simulink library "flexy_air_lib"  (R2020a)
settings: Solver=VariableStepAuto  StartTime=0.0  StopTime=10.0  RelTol=1e-3
settings Model: Creator=MK  LastModifiedBy=MK

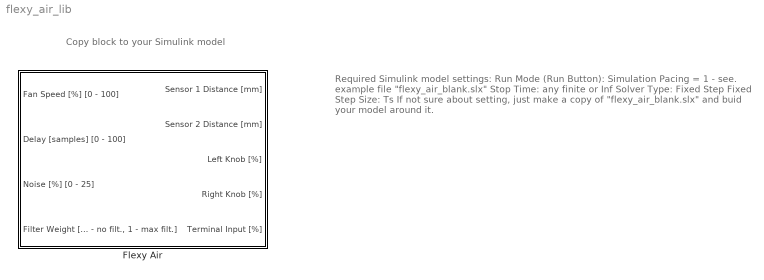
== system flexy_air_lib ==
  note: Copy block to your Simulink model
  note: Required Simulink model settings:
      |
      | Run Mode (Run Button): Simulation Pacing = 1 - see. example file "flexy_air_blank.slx"
      | Stop Time: any finite or Inf
      | Solver Type: Fixed Step
      | Fixed Step Size: Ts
      |
      | If not sure about setting, just make a copy of "flexy_air_blank.slx"
      | and buid your model around it.
  Flexy Air : Subsystem

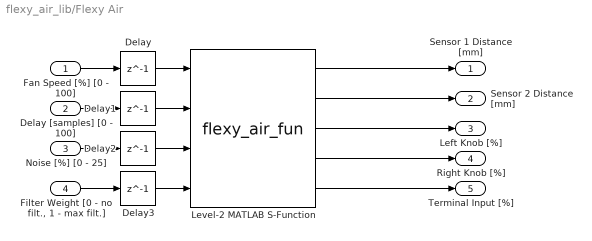
== system flexy_air_lib/Flexy Air ==
  Fan Speed [%] [0 - 100] : Inport
  Delay [samples] [0 - 100] : Inport  Port=2
  Noise [%] [0 - 25] : Inport  Port=3
  "Filter Weight [0 - no filt., 1 - max filt.]" : Inport  Port=4
  Delay{,1..3} (4 alike) : Delay  DelayLength=1
  Level-2 MATLAB S-Function : M-S-Function  FunctionName=flexy_air_fun  Parameters=Ts, Port, graceful_shutdown_opt
  Sensor 1 Distance [mm] : Outport
  Sensor 2 Distance [mm] : Outport  Port=2
  "Left Knob [%] " : Outport  Port=3
  "Right Knob [%] " : Outport  Port=4
  Terminal Input [%] : Outport  Port=5
  wires:
  Level-2 MATLAB S-Function/1 -> Sensor 1 Distance [mm]/1
  "Filter Weight [0 - no filt., 1 - max filt.]"/1 -> Delay3/1
  Level-2 MATLAB S-Function/5 -> Terminal Input [%]/1
  Delay [samples] [0 - 100]/1 -> Delay1/1
  Fan Speed [%] [0 - 100]/1 -> Delay/1
  Level-2 MATLAB S-Function/3 -> "Left Knob [%] "/1
  Noise [%] [0 - 25]/1 -> Delay2/1
  Level-2 MATLAB S-Function/4 -> "Right Knob [%] "/1
  Level-2 MATLAB S-Function/2 -> Sensor 2 Distance [mm]/1
  Delay/1 -> Level-2 MATLAB S-Function/1
  Delay1/1 -> Level-2 MATLAB S-Function/2
  Delay2/1 -> Level-2 MATLAB S-Function/3
  Delay3/1 -> Level-2 MATLAB S-Function/4
